simulink model "InvertedPendulum"  (R2014a)
settings: Solver=ode45  StartTime=0.0  StopTime=10.0  RelTol=1e-3
InitFcn:
  | Jeq = 1.84e-6
  | m = 0.0270
  | r = 0.0826
  | Kg = 1
  | Jm = 1.80e-4
  | ng = 1
  | nm = 0.69
  | L = 0.055
  | g = 9.8
  | Kt = 0.0334
  | R = 8.7
  | a = Jeq + m*r^2 + ng*kg^2*Jm
  | b = m*L*r
  | c = 4/3*m*L^2
  | d = m*g*L
  | f = (nm*ng*Kt*Kg)/R
settings Model: Creator=usmankhan  LastModifiedBy=usmankhan

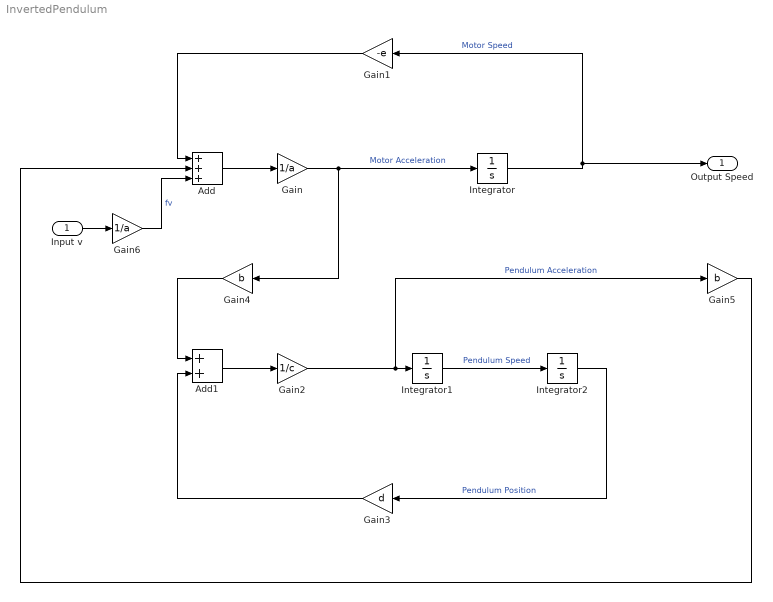
== system InvertedPendulum ==
  "Input v " : Inport
  Add : Sum  Inputs=+++
  Add1 : Sum
  Gain : Gain  Gain=1/a
  Gain1 : Gain  Gain=-e
  Gain2 : Gain  Gain=1/c
  Gain3 : Gain  Gain=d
  Gain4 : Gain  Gain=b
  Gain5 : Gain  Gain=b
  Gain6 : Gain  Gain=1/a
  Integrator : Integrator
  Integrator1 : Integrator
  Integrator2 : Integrator
  Output Speed : Outport
  wires:
  Add/1 -> Gain/1
  Gain/1 -> Gain4/1, Integrator/1  "Motor Acceleration"
  Integrator/1 -> Output Speed/1, Gain1/1  "Motor Speed"
  Gain1/1 -> Add/1
  Add1/1 -> Gain2/1
  Gain2/1 -> Gain5/1, Integrator1/1  "Pendulum Acceleration"
  Integrator1/1 -> Integrator2/1  "Pendulum Speed"
  Integrator2/1 -> Gain3/1  "Pendulum Position"
  Gain3/1 -> Add1/2
  Gain4/1 -> Add1/1
  Gain5/1 -> Add/2
  Gain6/1 -> Add/3  "fv"
  "Input v "/1 -> Gain6/1
